simulink model "RBFNN_1221"  (R2018a)
settings: Solver=FixedStepAuto  StartTime=0.0  StopTime=inf  FixedStep=0.001  RelTol=1e-3  EnableMultiTasking=on
undefined symbols (not defined in the file): HIL, j, qc_get_step_size
libraries: dsparch4 x28, quarc_library x17, simulink x7, vrlib x1
(part 3 of 6)

== matlab function RBFNN_1221/MATLAB Function7 ==
  data: p_end input; s output; v_max input; a_max input; ts input; t input; v output; a output; j output
function [s, v, a, j] = fcn(p_end, v_max, a_max, ts, t)
y=[0,0,0,0];

v_M=v_max;
a_M=a_max;

j_M	  = a_M*20.0;  % Max jerk (the rate of acceleration) is set as 20*Max acceleration */
delay = 3;       %output trajectory is set as zero in the peroid of delay */
freq  = 1.0/ts;    %sampling frequency/
pause =1;		%when the trajectory moves to zero position and final position, pause 1 sec */


% compute initial condition of each trajectory segment */
t0  = pause;
t1  = a_M/j_M; %加速度增大
t2  = v_M/a_M - a_M/j_M;%加速度不变
t3  = a_M/j_M;

a1 = j_M*t1;
a2 = a1;
a3 = a2 - j_M*t3;

v1 = j_M*t1*t1/2.0;
v2 = v1 + a1*t2;
v3 = v2 + a2*t3 - j_M*t3*t3/2.0;

s1 = j_M*t1*t1*t1/6;
s2 = s1 + v1*t2 + a1*t2*t2/2.0;
s3 = s2 + v2*t3 + a2*t3*t3/2.0 - j_M*t3*t3*t3/6.0;

t4  = (p_end - 2.0*s3)/v_M;
t5  = a_M/j_M;
t6  = v_M/a_M - a_M/j_M;
t7  = a_M/j_M;
t8  = pause;
t9  = pause;
t10 = a_M/j_M;
t11 = v_M/a_M - a_M/j_M;
t12 = a_M/j_M;
t13 = (p_end - 2.0*s3)/v_M;
t14 = a_M/j_M;
t15 = v_M/a_M - a_M/j_M;
t16 = a_M/j_M;
t17 = pause;

a4  = a3;
a5  = a4 - j_M*t5;
a6  = a5;
a7  = a6 + j_M*t7;
a8  = a7;
a9  = a8;
a10 = a9 - j_M*t10;
a11 = a10;
a12 = a11 + j_M*t12;
a13 = a12;
a14 = a13 + j_M*t14;
a15 = a14;

v4  = v3 + a3*t4;
v5  = v4 + a4*t5 - j_M*t5*t5/2.0;
v6  = v5 + a5*t6;
v7  = v6 + a6*t7 + j_M*t7*t7/2.0;
v8  = v7 + a7*t8;
v9  = v8 + a8*t9;
v10 = v9 + a9*t10 - j_M*t10*t10/2.0;
v11 = v10 + a10*t11;
v12 = v11 + a11*t12 + j_M*t12*t12/2.0;
v13 = v12 + a12*t13;
v14 = v13 + a13*t14 + j_M*t14*t14/2.0;
v15 = v14 + a14*t15;

s4  = s3 + v3*t4 + a3*t4*t4/2.0;
s5  = s4 + v4*t5 + a4*t5*t5/2.0 - j_M*t5*t5*t5/6.0;
s6  = s5 + v5*t6 + a5*t6*t6/2.0;
s7  = s6 + v6*t7 + a6*t7*t7/2.0 + j_M*t7*t7*t7/6.0;
s8  = s7 + v7*t8 + a7*t8*t8/2.0;
s9  = s8 + v8*t9 + a8*t9*t9/2.0;
s10 = s9 + v9*t10 + a9*t10*t10/2.0 - j_M*t10*t10*t10/6.0;
s11 = s10 + v10*t11 + a10*t11*t11/2.0;
s12 = s11 + v11*t12 + a11*t12*t12/2.0 + j_M*t12*t12*t12/6.0;
s13 = s12 + v12*t13 + a12*t13*t13/2.0;
s14 = s13 + v13*t14 + a13*t14*t14/2.0 + j_M*t14*t14*t14/6.0;
s15 = s14 + v14*t15 + a14*t15*t15/2.0;
s16 = s15 + v15*t16 + a15*t16*t16/2.0 - j_M*t16*t16*t16/6.0;

T0  = t0;
T1  = T0 + t1;
T2  = T1 + t2;
T3  = T2 + t3;
T4  = T3 + t4;
T5  = T4 + t5;
T6  = T5 + t6;
T7  = T6 + t7;
T8  = T7 + t8;
T9  = T8 + t9;
T10 = T9 + t10;
T11 = T10 + t11;
T12 = T11 + t12;
T13 = T12 + t13;
T14 = T13 + t14;
T15 = T14 + t15;
T16 = T15 + t16;
T17 = T16 + t17;

%/* generate trajectory */
if(t<=delay)
    y(4) = 0.0;	   % /* jerk */
    y(2) = 0.0;		%/* acceleration */
    y(3) = 0.0;		%/* velocity */
    y(1) = 0.0;		%/* position */
else
    % 	 q0	  = *uPtrs[0];%q0 is what?
    T	  = T17*freq;
    tt   = (t-delay)*freq;
    rt   = mod(tt,T);
    rrt  = rt/freq;
    
    if(rt<=T0*freq)
        y(4) = 0.0;	   % /* jerk */
        y(3) = 0.0;		%/* acceleration */
        y(2) = 0.0;		%/* velocity */
        y(1) = 0.0;		%/* position */
    end
    
    if(rt>T0*freq && rt<=T1*freq)
        y(4) = j_M;
        y(3) = j_M*(rrt-T0);
        y(2) = j_M*(rrt-T0)*(rrt-T0)/2.0;
        y(1) = j_M*(rrt-T0)*(rrt-T0)*(rrt-T0)/6.0;
    end
    
    
    if(rt>T1*freq && rt<=T2*freq)
        y(4) = 0.0;
        y(3) = a1;
        y(2) = v1 + a1*(rrt-T1);
        y(1) = s1 + v1*(rrt-T1) + a1*(rrt-T1)*(rrt-T1)/2.0;
    end
    
    
    if(rt>T2*freq && rt<=T3*freq)
        y(4) = -j_M;
        y(3) = a2 - j_M*(rrt-T2);
        y(2) = v2 + a2*(rrt-T2) - j_M*(rrt-T2)*(rrt-T2)/2.0;
        y(1) = s2 + v2*(rrt-T2) + a2*(rrt-T2)*(rrt-T2)/2.0 - j_M*(rrt-T2)*(rrt-T2)*(rrt-T2)/6.0;
    end
    
    
    if(rt>T3*freq && rt<=T4*freq)
        y(4) = 0.0;
        y(3) = a3;
        y(2) = v3 + a3*(rrt-T3);
        y(1) = s3 + v3*(rrt-T3) + a3*(rrt-T3)*(rrt-T3)/2.0;
    end
    
    
    if(rt>T4*freq && rt<=T5*freq)
        y(4) = -j_M;
        y(3) = a4 - j_M*(rrt-T4);
        y(2) = v4 + a4*(rrt-T4) - j_M*(rrt-T4)*(rrt-T4)/2.0;
        y(1) = s4 + v4*(rrt-T4) + a4*(rrt-T4)*(rrt-T4)/2.0 - j_M*(rrt-T4)*(rrt-T4)*(rrt-T4)/6.0;
    end
    
    
    if(rt>T5*freq && rt<=T6*freq)
        y(4) = 0;
        y(3) = a5;
        y(2) = v5 + a5*(rrt-T5);
        y(1) = s5 + v5*(rrt-T5) + a5*(rrt-T5)*(rrt-T5)/2.0;
    end
    
    
    if(rt>T6*freq && rt<=T7*freq)
        y(4) = j_M;
        y(3) = a6 + j_M*(rrt-T6);
        y(2) = v6 + a6*(rrt-T6) + j_M*(rrt-T6)*(rrt-T6)/2.0;
        y(1) = s6 + v6*(rrt-T6) + a6*(rrt-T6)*(rrt-T6)/2.0 + j_M*(rrt-T6)*(rrt-T6)*(rrt-T6)/6.0;
    end
    
    
    if(rt>T7*freq && rt<=T8*freq)
        y(4) = 0.0;
        y(3) = 0.0;
        y(2) = 0.0;
        y(1) = s7;
    end
    
    
    if(rt>T8*freq && rt<=T9*freq)
        y(4) = 0.0;
        y(3) = 0.0;
        y(2) = 0.0;
        y(1) = s8;
    end
    
    
    if(rt>T9*freq && rt<=T10*freq)
        y(4) = -j_M;
        y(3) = a9 - j_M*(rrt-T9);
        y(2) = v9 + a9*(rrt-T9) - j_M*(rrt-T9)*(rrt-T9)/2.0;
        y(1) = s9 + v9*(rrt-T9) + a9*(rrt-T9)*(rrt-T9)/2.0 - j_M*(rrt-T9)*(rrt-T9)*(rrt-T9)/6.0;
    end
    
    
    if(rt>T10*freq && rt<=T11*freq)
        y(4) = 0.0;
        y(3) = a10;
        y(2) = v10 + a10*(rrt-T10);
        y(1) = s10 + v10*(rrt-T10) + a10*(rrt-T10)*(rrt-T10)/2.0;
    end
    
    
    
    if(rt>T11*freq && rt<=T12*freq)
        y(4) = j_M;
        y(3) = a11 + j_M*(rrt-T11);
        y(2) = v11 + a11*(rrt-T11) + j_M*(rrt-T11)*(rrt-T11)/2.0;
        y(1) = s11 + v11*(rrt-T11) + a11*(rrt-T11)*(rrt-T11)/2.0 + j_M*(rrt-T11)*(rrt-T11)*(rrt-T11)/6.0;
    end
    
    
    if(rt>T12*freq && rt<=T13*freq)
        y(4) = 0;
        y(3) = a12;
        y(2) = v12 + a12*(rrt-T12);
        y(1) = s12 + v12*(rrt-T12) + a12*(rrt-T12)*(rrt-T12)/2.0;
    end
    
    
    if(rt>T13*freq && rt<=T14*freq)
        y(4) = j_M;
        y(3) = a13 + j_M*(rrt-T13);
        y(2) = v13 + a13*(rrt-T13) + j_M*(rrt-T13)*(rrt-T13)/2.0;
        y(1) = s13 + v13*(rrt-T13) + a13*(rrt-T13)*(rrt-T13)/2.0 + j_M*(rrt-T13)*(rrt-T13)*(rrt-T13)/6.0;
    end
    
    
    if(rt>T14*freq && rt<=T15*freq)
        y(4) = 0.0;
        y(3) = a14;
        y(2) = v14 + a14*(rrt-T14);
        y(1) = s14 + v14*(rrt-T14) + a14*(rrt-T14)*(rrt-T14)/2.0;
    end
    
    
    if(rt>T15*freq && rt<=T16*freq)
        y(4) = -j_M;
        y(3) = a15 - j_M*(rrt-T15);
        y(2) = v15 + a15*(rrt-T15) - j_M*(rrt-T15)*(rrt-T15)/2.0;
        y(1) = s15 + v15*(rrt-T15) + a15*(rrt-T15)*(rrt-T15)/2.0 - j_M*(rrt-T15)*(rrt-T15)*(rrt-T15)/6.0;
    end
    
    
    if(rt>T16*freq && rt<=T17*freq)
        y(4) = 0.0;
        y(3) = 0.0;
        y(2) = 0.0;
        y(1) = s16;
    end
end
s = y(1);
v = y(2);
a = y(3);
j = y(4);

== matlab function RBFNN_1221/Obs Para Generator3 ==
  data: a input; gain input; k_obs output; th input
function k_obs = fcn(a, gain, th)

if a <= th
    b = 22.5*a-37.5;
else
    b = 31.16*a - 68.8; % a>=2.5
end
k_obs  = ([1 1/a 1/b] .* gain.^[1 2 3])';

== matlab function RBFNN_1221/Subsystem9/MATLAB Function1 ==
  data: x input; u input; y output
function y = fcn(x,u)
y=u(x);
end

== matlab function RBFNN_1221/MATLAB Function8 ==
  data: p_end input; s output; v_max input; a_max input; ts input; t input; v output; a output; j output
function [s, v, a, j] = fcn(p_end, v_max, a_max, ts, t)
y=[0,0,0,0];

v_M=v_max;
a_M=a_max;

j_M	  = a_M*20.0;  % Max jerk (the rate of acceleration) is set as 20*Max acceleration */
delay = 3;       %output trajectory is set as zero in the peroid of delay */
freq  = 1.0/ts;    %sampling frequency/
pause =1;		%when the trajectory moves to zero position and final position, pause 1 sec */


% compute initial condition of each trajectory segment */
t0  = pause;
t1  = a_M/j_M; %加速度增大
t2  = v_M/a_M - a_M/j_M;%加速度不变
t3  = a_M/j_M;

a1 = j_M*t1;
a2 = a1;
a3 = a2 - j_M*t3;

v1 = j_M*t1*t1/2.0;
v2 = v1 + a1*t2;
v3 = v2 + a2*t3 - j_M*t3*t3/2.0;

s1 = j_M*t1*t1*t1/6;
s2 = s1 + v1*t2 + a1*t2*t2/2.0;
s3 = s2 + v2*t3 + a2*t3*t3/2.0 - j_M*t3*t3*t3/6.0;

t4  = (p_end - 2.0*s3)/v_M;
t5  = a_M/j_M;
t6  = v_M/a_M - a_M/j_M;
t7  = a_M/j_M;
t8  = pause;
t9  = pause;
t10 = a_M/j_M;
t11 = v_M/a_M - a_M/j_M;
t12 = a_M/j_M;
t13 = (p_end - 2.0*s3)/v_M;
t14 = a_M/j_M;
t15 = v_M/a_M - a_M/j_M;
t16 = a_M/j_M;
t17 = pause;

a4  = a3;
a5  = a4 - j_M*t5;
a6  = a5;
a7  = a6 + j_M*t7;
a8  = a7;
a9  = a8;
a10 = a9 - j_M*t10;
a11 = a10;
a12 = a11 + j_M*t12;
a13 = a12;
a14 = a13 + j_M*t14;
a15 = a14;

v4  = v3 + a3*t4;
v5  = v4 + a4*t5 - j_M*t5*t5/2.0;
v6  = v5 + a5*t6;
v7  = v6 + a6*t7 + j_M*t7*t7/2.0;
v8  = v7 + a7*t8;
v9  = v8 + a8*t9;
v10 = v9 + a9*t10 - j_M*t10*t10/2.0;
v11 = v10 + a10*t11;
v12 = v11 + a11*t12 + j_M*t12*t12/2.0;
v13 = v12 + a12*t13;
v14 = v13 + a13*t14 + j_M*t14*t14/2.0;
v15 = v14 + a14*t15;

s4  = s3 + v3*t4 + a3*t4*t4/2.0;
s5  = s4 + v4*t5 + a4*t5*t5/2.0 - j_M*t5*t5*t5/6.0;
s6  = s5 + v5*t6 + a5*t6*t6/2.0;
s7  = s6 + v6*t7 + a6*t7*t7/2.0 + j_M*t7*t7*t7/6.0;
s8  = s7 + v7*t8 + a7*t8*t8/2.0;
s9  = s8 + v8*t9 + a8*t9*t9/2.0;
s10 = s9 + v9*t10 + a9*t10*t10/2.0 - j_M*t10*t10*t10/6.0;
s11 = s10 + v10*t11 + a10*t11*t11/2.0;
s12 = s11 + v11*t12 + a11*t12*t12/2.0 + j_M*t12*t12*t12/6.0;
s13 = s12 + v12*t13 + a12*t13*t13/2.0;
s14 = s13 + v13*t14 + a13*t14*t14/2.0 + j_M*t14*t14*t14/6.0;
s15 = s14 + v14*t15 + a14*t15*t15/2.0;
s16 = s15 + v15*t16 + a15*t16*t16/2.0 - j_M*t16*t16*t16/6.0;

T0  = t0;
T1  = T0 + t1;
T2  = T1 + t2;
T3  = T2 + t3;
T4  = T3 + t4;
T5  = T4 + t5;
T6  = T5 + t6;
T7  = T6 + t7;
T8  = T7 + t8;
T9  = T8 + t9;
T10 = T9 + t10;
T11 = T10 + t11;
T12 = T11 + t12;
T13 = T12 + t13;
T14 = T13 + t14;
T15 = T14 + t15;
T16 = T15 + t16;
T17 = T16 + t17;

%/* generate trajectory */
if(t<=delay)
    y(4) = 0.0;	   % /* jerk */
    y(2) = 0.0;		%/* acceleration */
    y(3) = 0.0;		%/* velocity */
    y(1) = 0.0;		%/* position */
else
    % 	 q0	  = *uPtrs[0];%q0 is what?
    T	  = T17*freq;
    tt   = (t-delay)*freq;
    rt   = mod(tt,T);
    rrt  = rt/freq;
    
    if(rt<=T0*freq)
        y(4) = 0.0;	   % /* jerk */
        y(3) = 0.0;		%/* acceleration */
        y(2) = 0.0;		%/* velocity */
        y(1) = 0.0;		%/* position */
    end
    
    if(rt>T0*freq && rt<=T1*freq)
        y(4) = j_M;
        y(3) = j_M*(rrt-T0);
        y(2) = j_M*(rrt-T0)*(rrt-T0)/2.0;
        y(1) = j_M*(rrt-T0)*(rrt-T0)*(rrt-T0)/6.0;
    end
    
    
    if(rt>T1*freq && rt<=T2*freq)
        y(4) = 0.0;
        y(3) = a1;
        y(2) = v1 + a1*(rrt-T1);
        y(1) = s1 + v1*(rrt-T1) + a1*(rrt-T1)*(rrt-T1)/2.0;
    end
    
    
    if(rt>T2*freq && rt<=T3*freq)
        y(4) = -j_M;
        y(3) = a2 - j_M*(rrt-T2);
        y(2) = v2 + a2*(rrt-T2) - j_M*(rrt-T2)*(rrt-T2)/2.0;
        y(1) = s2 + v2*(rrt-T2) + a2*(rrt-T2)*(rrt-T2)/2.0 - j_M*(rrt-T2)*(rrt-T2)*(rrt-T2)/6.0;
    end
    
    
    if(rt>T3*freq && rt<=T4*freq)
        y(4) = 0.0;
        y(3) = a3;
        y(2) = v3 + a3*(rrt-T3);
        y(1) = s3 + v3*(rrt-T3) + a3*(rrt-T3)*(rrt-T3)/2.0;
    end
    
    
    if(rt>T4*freq && rt<=T5*freq)
        y(4) = -j_M;
        y(3) = a4 - j_M*(rrt-T4);
        y(2) = v4 + a4*(rrt-T4) - j_M*(rrt-T4)*(rrt-T4)/2.0;
        y(1) = s4 + v4*(rrt-T4) + a4*(rrt-T4)*(rrt-T4)/2.0 - j_M*(rrt-T4)*(rrt-T4)*(rrt-T4)/6.0;
    end
    
    
    if(rt>T5*freq && rt<=T6*freq)
        y(4) = 0;
        y(3) = a5;
        y(2) = v5 + a5*(rrt-T5);
        y(1) = s5 + v5*(rrt-T5) + a5*(rrt-T5)*(rrt-T5)/2.0;
    end
    
    
    if(rt>T6*freq && rt<=T7*freq)
        y(4) = j_M;
        y(3) = a6 + j_M*(rrt-T6);
        y(2) = v6 + a6*(rrt-T6) + j_M*(rrt-T6)*(rrt-T6)/2.0;
        y(1) = s6 + v6*(rrt-T6) + a6*(rrt-T6)*(rrt-T6)/2.0 + j_M*(rrt-T6)*(rrt-T6)*(rrt-T6)/6.0;
    end
    
    
    if(rt>T7*freq && rt<=T8*freq)
        y(4) = 0.0;
        y(3) = 0.0;
        y(2) = 0.0;
        y(1) = s7;
    end
    
    
    if(rt>T8*freq && rt<=T9*freq)
        y(4) = 0.0;
        y(3) = 0.0;
        y(2) = 0.0;
        y(1) = s8;
    end
    
    
    if(rt>T9*freq && rt<=T10*freq)
        y(4) = -j_M;
        y(3) = a9 - j_M*(rrt-T9);
        y(2) = v9 + a9*(rrt-T9) - j_M*(rrt-T9)*(rrt-T9)/2.0;
        y(1) = s9 + v9*(rrt-T9) + a9*(rrt-T9)*(rrt-T9)/2.0 - j_M*(rrt-T9)*(rrt-T9)*(rrt-T9)/6.0;
    end
    
    
    if(rt>T10*freq && rt<=T11*freq)
        y(4) = 0.0;
        y(3) = a10;
        y(2) = v10 + a10*(rrt-T10);
        y(1) = s10 + v10*(rrt-T10) + a10*(rrt-T10)*(rrt-T10)/2.0;
    end
    
    
    
    if(rt>T11*freq && rt<=T12*freq)
        y(4) = j_M;
        y(3) = a11 + j_M*(rrt-T11);
        y(2) = v11 + a11*(rrt-T11) + j_M*(rrt-T11)*(rrt-T11)/2.0;
        y(1) = s11 + v11*(rrt-T11) + a11*(rrt-T11)*(rrt-T11)/2.0 + j_M*(rrt-T11)*(rrt-T11)*(rrt-T11)/6.0;
    end
    
    
    if(rt>T12*freq && rt<=T13*freq)
        y(4) = 0;
        y(3) = a12;
        y(2) = v12 + a12*(rrt-T12);
        y(1) = s12 + v12*(rrt-T12) + a12*(rrt-T12)*(rrt-T12)/2.0;
    end
    
    
    if(rt>T13*freq && rt<=T14*freq)
        y(4) = j_M;
        y(3) = a13 + j_M*(rrt-T13);
        y(2) = v13 + a13*(rrt-T13) + j_M*(rrt-T13)*(rrt-T13)/2.0;
        y(1) = s13 + v13*(rrt-T13) + a13*(rrt-T13)*(rrt-T13)/2.0 + j_M*(rrt-T13)*(rrt-T13)*(rrt-T13)/6.0;
    end
    
    
    if(rt>T14*freq && rt<=T15*freq)
        y(4) = 0.0;
        y(3) = a14;
        y(2) = v14 + a14*(rrt-T14);
        y(1) = s14 + v14*(rrt-T14) + a14*(rrt-T14)*(rrt-T14)/2.0;
    end
    
    
    if(rt>T15*freq && rt<=T16*freq)
        y(4) = -j_M;
        y(3) = a15 - j_M*(rrt-T15);
        y(2) = v15 + a15*(rrt-T15) - j_M*(rrt-T15)*(rrt-T15)/2.0;
        y(1) = s15 + v15*(rrt-T15) + a15*(rrt-T15)*(rrt-T15)/2.0 - j_M*(rrt-T15)*(rrt-T15)*(rrt-T15)/6.0;
    end
    
    
    if(rt>T16*freq && rt<=T17*freq)
        y(4) = 0.0;
        y(3) = 0.0;
        y(2) = 0.0;
        y(1) = s16;
    end
end
s = y(1);
v = y(2);
a = y(3);
j = y(4);

== matlab function RBFNN_1221/limit_u2 ==
  data: u input; y output
function y = fcn(u)
y=u;
if u>10
    y=10;
end
if u<-10
    y=-10;
end
end

== matlab function RBFNN_1221/MATLAB Function1 ==
  data: bias input; out output; xv input
function out = fcn(bias,xv)
out = xv;
if xv > 0
    out = xv + bias;
end
if xv < 0
    out = xv - bias;
end
end

== matlab function RBFNN_1221/Obs Para Generator4 ==
  data: a input; gain input; k_obs output; th input
function k_obs = fcn(a, gain, th)

if a <= th
    b = 22.5*a-37.5;
else
    b = 31.16*a - 68.8; % a>=2.5
end
k_obs  = ([1 1/a 1/b] .* gain.^[1 2 3])';

== matlab function RBFNN_1221/MATLAB Function9 ==
  data: p_end input; s output; v_max input; a_max input; ts input; t input; v output; a output; j output
function [s, v, a, j] = fcn(p_end, v_max, a_max, ts, t)
y=[0,0,0,0];

v_M=v_max;
a_M=a_max;

j_M	  = a_M*20.0;  % Max jerk (the rate of acceleration) is set as 20*Max acceleration */
delay = 3;       %output trajectory is set as zero in the peroid of delay */
freq  = 1.0/ts;    %sampling frequency/
pause =1;		%when the trajectory moves to zero position and final position, pause 1 sec */


% compute initial condition of each trajectory segment */
t0  = pause;
t1  = a_M/j_M; %加速度增大
t2  = v_M/a_M - a_M/j_M;%加速度不变
t3  = a_M/j_M;

a1 = j_M*t1;
a2 = a1;
a3 = a2 - j_M*t3;

v1 = j_M*t1*t1/2.0;
v2 = v1 + a1*t2;
v3 = v2 + a2*t3 - j_M*t3*t3/2.0;

s1 = j_M*t1*t1*t1/6;
s2 = s1 + v1*t2 + a1*t2*t2/2.0;
s3 = s2 + v2*t3 + a2*t3*t3/2.0 - j_M*t3*t3*t3/6.0;

t4  = (p_end - 2.0*s3)/v_M;
t5  = a_M/j_M;
t6  = v_M/a_M - a_M/j_M;
t7  = a_M/j_M;
t8  = pause;
t9  = pause;
t10 = a_M/j_M;
t11 = v_M/a_M - a_M/j_M;
t12 = a_M/j_M;
t13 = (p_end - 2.0*s3)/v_M;
t14 = a_M/j_M;
t15 = v_M/a_M - a_M/j_M;
t16 = a_M/j_M;
t17 = pause;

a4  = a3;
a5  = a4 - j_M*t5;
a6  = a5;
a7  = a6 + j_M*t7;
a8  = a7;
a9  = a8;
a10 = a9 - j_M*t10;
a11 = a10;
a12 = a11 + j_M*t12;
a13 = a12;
a14 = a13 + j_M*t14;
a15 = a14;

v4  = v3 + a3*t4;
v5  = v4 + a4*t5 - j_M*t5*t5/2.0;
v6  = v5 + a5*t6;
v7  = v6 + a6*t7 + j_M*t7*t7/2.0;
v8  = v7 + a7*t8;
v9  = v8 + a8*t9;
v10 = v9 + a9*t10 - j_M*t10*t10/2.0;
v11 = v10 + a10*t11;
v12 = v11 + a11*t12 + j_M*t12*t12/2.0;
v13 = v12 + a12*t13;
v14 = v13 + a13*t14 + j_M*t14*t14/2.0;
v15 = v14 + a14*t15;

s4  = s3 + v3*t4 + a3*t4*t4/2.0;
s5  = s4 + v4*t5 + a4*t5*t5/2.0 - j_M*t5*t5*t5/6.0;
s6  = s5 + v5*t6 + a5*t6*t6/2.0;
s7  = s6 + v6*t7 + a6*t7*t7/2.0 + j_M*t7*t7*t7/6.0;
s8  = s7 + v7*t8 + a7*t8*t8/2.0;
s9  = s8 + v8*t9 + a8*t9*t9/2.0;
s10 = s9 + v9*t10 + a9*t10*t10/2.0 - j_M*t10*t10*t10/6.0;
s11 = s10 + v10*t11 + a10*t11*t11/2.0;
s12 = s11 + v11*t12 + a11*t12*t12/2.0 + j_M*t12*t12*t12/6.0;
s13 = s12 + v12*t13 + a12*t13*t13/2.0;
s14 = s13 + v13*t14 + a13*t14*t14/2.0 + j_M*t14*t14*t14/6.0;
s15 = s14 + v14*t15 + a14*t15*t15/2.0;
s16 = s15 + v15*t16 + a15*t16*t16/2.0 - j_M*t16*t16*t16/6.0;

T0  = t0;
T1  = T0 + t1;
T2  = T1 + t2;
T3  = T2 + t3;
T4  = T3 + t4;
T5  = T4 + t5;
T6  = T5 + t6;
T7  = T6 + t7;
T8  = T7 + t8;
T9  = T8 + t9;
T10 = T9 + t10;
T11 = T10 + t11;
T12 = T11 + t12;
T13 = T12 + t13;
T14 = T13 + t14;
T15 = T14 + t15;
T16 = T15 + t16;
T17 = T16 + t17;

%/* generate trajectory */
if(t<=delay)
    y(4) = 0.0;	   % /* jerk */
    y(2) = 0.0;		%/* acceleration */
    y(3) = 0.0;		%/* velocity */
    y(1) = 0.0;		%/* position */
else
    % 	 q0	  = *uPtrs[0];%q0 is what?
    T	  = T17*freq;
    tt   = (t-delay)*freq;
    rt   = mod(tt,T);
    rrt  = rt/freq;
    
    if(rt<=T0*freq)
        y(4) = 0.0;	   % /* jerk */
        y(3) = 0.0;		%/* acceleration */
        y(2) = 0.0;		%/* velocity */
        y(1) = 0.0;		%/* position */
    end
    
    if(rt>T0*freq && rt<=T1*freq)
        y(4) = j_M;
        y(3) = j_M*(rrt-T0);
        y(2) = j_M*(rrt-T0)*(rrt-T0)/2.0;
        y(1) = j_M*(rrt-T0)*(rrt-T0)*(rrt-T0)/6.0;
    end
    
    
    if(rt>T1*freq && rt<=T2*freq)
        y(4) = 0.0;
        y(3) = a1;
        y(2) = v1 + a1*(rrt-T1);
        y(1) = s1 + v1*(rrt-T1) + a1*(rrt-T1)*(rrt-T1)/2.0;
    end
    
    
    if(rt>T2*freq && rt<=T3*freq)
        y(4) = -j_M;
        y(3) = a2 - j_M*(rrt-T2);
        y(2) = v2 + a2*(rrt-T2) - j_M*(rrt-T2)*(rrt-T2)/2.0;
        y(1) = s2 + v2*(rrt-T2) + a2*(rrt-T2)*(rrt-T2)/2.0 - j_M*(rrt-T2)*(rrt-T2)*(rrt-T2)/6.0;
    end
    
    
    if(rt>T3*freq && rt<=T4*freq)
        y(4) = 0.0;
        y(3) = a3;
        y(2) = v3 + a3*(rrt-T3);
        y(1) = s3 + v3*(rrt-T3) + a3*(rrt-T3)*(rrt-T3)/2.0;
    end
    
    
    if(rt>T4*freq && rt<=T5*freq)
        y(4) = -j_M;
        y(3) = a4 - j_M*(rrt-T4);
        y(2) = v4 + a4*(rrt-T4) - j_M*(rrt-T4)*(rrt-T4)/2.0;
        y(1) = s4 + v4*(rrt-T4) + a4*(rrt-T4)*(rrt-T4)/2.0 - j_M*(rrt-T4)*(rrt-T4)*(rrt-T4)/6.0;
    end
    
    
    if(rt>T5*freq && rt<=T6*freq)
        y(4) = 0;
        y(3) = a5;
        y(2) = v5 + a5*(rrt-T5);
        y(1) = s5 + v5*(rrt-T5) + a5*(rrt-T5)*(rrt-T5)/2.0;
    end
    
    
    if(rt>T6*freq && rt<=T7*freq)
        y(4) = j_M;
        y(3) = a6 + j_M*(rrt-T6);
        y(2) = v6 + a6*(rrt-T6) + j_M*(rrt-T6)*(rrt-T6)/2.0;
        y(1) = s6 + v6*(rrt-T6) + a6*(rrt-T6)*(rrt-T6)/2.0 + j_M*(rrt-T6)*(rrt-T6)*(rrt-T6)/6.0;
    end
    
    
    if(rt>T7*freq && rt<=T8*freq)
        y(4) = 0.0;
        y(3) = 0.0;
        y(2) = 0.0;
        y(1) = s7;
    end
    
    
    if(rt>T8*freq && rt<=T9*freq)
        y(4) = 0.0;
        y(3) = 0.0;
        y(2) = 0.0;
        y(1) = s8;
    end
    
    
    if(rt>T9*freq && rt<=T10*freq)
        y(4) = -j_M;
        y(3) = a9 - j_M*(rrt-T9);
        y(2) = v9 + a9*(rrt-T9) - j_M*(rrt-T9)*(rrt-T9)/2.0;
        y(1) = s9 + v9*(rrt-T9) + a9*(rrt-T9)*(rrt-T9)/2.0 - j_M*(rrt-T9)*(rrt-T9)*(rrt-T9)/6.0;
    end
    
    
    if(rt>T10*freq && rt<=T11*freq)
        y(4) = 0.0;
        y(3) = a10;
        y(2) = v10 + a10*(rrt-T10);
        y(1) = s10 + v10*(rrt-T10) + a10*(rrt-T10)*(rrt-T10)/2.0;
    end
    
    
    
    if(rt>T11*freq && rt<=T12*freq)
        y(4) = j_M;
        y(3) = a11 + j_M*(rrt-T11);
        y(2) = v11 + a11*(rrt-T11) + j_M*(rrt-T11)*(rrt-T11)/2.0;
        y(1) = s11 + v11*(rrt-T11) + a11*(rrt-T11)*(rrt-T11)/2.0 + j_M*(rrt-T11)*(rrt-T11)*(rrt-T11)/6.0;
    end
    
    
    if(rt>T12*freq && rt<=T13*freq)
        y(4) = 0;
        y(3) = a12;
        y(2) = v12 + a12*(rrt-T12);
        y(1) = s12 + v12*(rrt-T12) + a12*(rrt-T12)*(rrt-T12)/2.0;
    end
    
    
    if(rt>T13*freq && rt<=T14*freq)
        y(4) = j_M;
        y(3) = a13 + j_M*(rrt-T13);
        y(2) = v13 + a13*(rrt-T13) + j_M*(rrt-T13)*(rrt-T13)/2.0;
        y(1) = s13 + v13*(rrt-T13) + a13*(rrt-T13)*(rrt-T13)/2.0 + j_M*(rrt-T13)*(rrt-T13)*(rrt-T13)/6.0;
    end
    
    
    if(rt>T14*freq && rt<=T15*freq)
        y(4) = 0.0;
        y(3) = a14;
        y(2) = v14 + a14*(rrt-T14);
        y(1) = s14 + v14*(rrt-T14) + a14*(rrt-T14)*(rrt-T14)/2.0;
    end
    
    
    if(rt>T15*freq && rt<=T16*freq)
        y(4) = -j_M;
        y(3) = a15 - j_M*(rrt-T15);
        y(2) = v15 + a15*(rrt-T15) - j_M*(rrt-T15)*(rrt-T15)/2.0;
        y(1) = s15 + v15*(rrt-T15) + a15*(rrt-T15)*(rrt-T15)/2.0 - j_M*(rrt-T15)*(rrt-T15)*(rrt-T15)/6.0;
    end
    
    
    if(rt>T16*freq && rt<=T17*freq)
        y(4) = 0.0;
        y(3) = 0.0;
        y(2) = 0.0;
        y(1) = s16;
    end
end
s = y(1);
v = y(2);
a = y(3);
j = y(4);

== matlab function RBFNN_1221/limit_u3 ==
  data: u input; y output
function y = fcn(u)
y=u;
if u>10
    y=10;
end
if u<-10
    y=-10;
end
end

== matlab function RBFNN_1221/Subsystem8/Enabled Subsystem/Round Traj Planner ==
  data: p_center input; p_round output size=[3,1]; v_normal input; radius input; theta input; v_toward input; q_round output size=[4 1]; err output size=1
function [p_round, q_round, err] = fcn(p_center, v_normal, radius, theta, v_toward)

temp = atan2(-v_normal(3),v_normal(1));
v_init_r = [sin(temp),0,cos(temp)];
v_orth = cross(v_normal, v_init_r);
p_round = p_center + radius * (v_init_r'.*cos(theta) + v_orth.'*sin(theta));
q_round = InvKin(v_toward, p_round);

err = 0;
if max(abs(imag(q_round))~=0)
	err = err+1;
elseif isnan(sum(q_round))
	err = err+2;
end

== matlab function RBFNN_1221/Subsystem9/MATLAB Function ==
  data: Xcenter input; Ycenter input; height1 input; traj output size=[1 3]; height2 input; scale_factor input; span input; phase input; phase_last input; phase_start_time_last input; time input; phase_start_time output; err output
% ZJU形状轨迹生成
% 
% height1：书写高度
% height2：抬起高度

function [traj, phase_start_time, err] = fcn(Xcenter, Ycenter, height1, height2, scale_factor, span, phase, phase_last, phase_start_time_last, time)

% 平移缩放
% Traj_Z = [3.48433829875678,35.4885053891162;5.19457971416122,35.5831283413590;7.07593708942604,35.6227938555666;9.01422182304440,35.7222247489255;11.1233721029233,35.9423883858658;12.6056536713138,35.9736400031203;14.4300002170251,36.0121035320489;15.7412492967551,36.0397491934664;16.9954875469317,36.0661928696048;18.4209252281685,35.9791157138358;19.7320073654987,36.1238881629977;20.8151296558149,36.2052892771713;22.0122736052380,36.2890943619029;23.4945551736285,36.3203459791574;24.8628150829120,36.3491936258538;25.9460208444281,36.3720313461552;26.0030316739815,36.3732333314342;26.0030316739815,36.3732333314342;26.0030316739815,36.3732333314342;24.8647349205104,35.0022355667930;24.0114923148066,33.6372477285468;23.4995634456244,32.8065423468247;22.8165186165817,32.0307944031377;22.0201198980316,30.7841353379149;21.1101168763742,29.2422553327731;20.3141355138237,27.7027792981893;19.5175698528737,26.5732470207110;18.4365343425558,25.0277610597321;17.6400521528057,23.8396653883816;16.6725374743952,22.6479637611940;15.8192113974915,21.3415393168201;14.7375915887741,20.2059971129467;13.7698264967638,19.1899856673758;12.6312793296929,17.9946780843511;11.8923087966959,16.4564040350464;10.8106889879785,15.3208618311730;10.0138729134287,14.3670197353113;9.50202751544635,13.4777509597169;8.02174925585426,12.0409778895293;7.33953913881094,10.6795960071202;6.20132585653972,9.25003484860675;5.23439547652874,7.64838946431369;4.43791328677867,6.46029379296318;3.18551140300062,5.14545545163609;3.24293958855376,4.85384046755404;3.41405554841413,4.79888302951889;3.52807720752109,4.80128700007692;3.58508803707457,4.80248898535594;3.64209886662805,4.80369097063496;5.18130779337206,4.89470796704069;6.77744407846961,5.04549034259766;7.68953388012534,5.12328550093417;8.88659435834854,5.26565397953800;10.4828141146460,5.35787296122275;12.3069937179575,5.51346327789579;13.2762612915666,5.47533363376691;14.6445212008501,5.50418128046337;16.5826389920686,5.72073896156666;18.0651709740588,5.57630039720452;19.6614742015562,5.60995598501705;21.7137805942816,5.71179084893396;23.4808658968396,5.92474257420019;25.1914411970438,5.78511195095413;27.0157877427551,5.82357547988274;27.1296424594622,5.94310623818520;27.2439980033689,5.71125663325439];
% Traj_U = [72.6379737199274,37.2978938957997;72.5256214848191,36.1242220477974;72.5270404952180,35.1286443519698;72.4151056161093,33.6621555346065;72.2455756090476,32.6044084890696;72.5317148824142,31.8490942951259;72.4764569480592,30.6180610385304;72.4777924872581,29.6810467365751;72.4797123248566,28.3340886775142;72.4810478640555,27.3970743755588;72.4827172880541,26.2258064981145;72.4853883664519,24.3517778942037;72.5447363896035,22.7132048510608;72.7753673150153,20.9025475821383;72.7767863254142,19.9069698863107;72.8924774085198,18.7381059794245;72.8941468325184,17.5668381019802;72.8956493141172,16.5126970122804;73.0111734548229,15.4609598931386;73.4120021568958,14.2395425187753;73.6411306007089,13.4830263395526;74.0412915331823,12.7301161161670;74.4414524656558,11.9772058927814;75.0127293579896,11.1693382313606;75.5270788919699,10.3017051907886;75.9268224684437,9.84161193676402;76.9540190548055,9.16048694531982;77.8099327389071,8.65144617965519;78.6657629518088,8.20096880786279;79.4648327487567,7.57359926917472;80.4347680919653,7.06696247406814;81.5753185678346,6.85674860415967;82.2026881065226,6.69428026061224;83.2858938680387,6.71711798091361;84.3690996295549,6.73995570121497;85.6233378797314,6.76639937735339;87.3331619391362,7.15383929895724;88.9280461562348,8.18307258259739;89.8964790178445,8.73057687719062;90.5793569044873,9.62345160862204;91.6614775404043,10.4076134492622;92.7432642915215,11.4260288653911;93.0844945568431,12.0188747157874;93.5956721852260,13.3766506423594;93.5940862324273,14.4893551259315;93.5922498660288,15.7777497911201;93.6467565595843,17.5358535925655;93.7011797819399,19.3525207878831;93.6998442427410,20.2895350898385;93.6404962195894,21.9281081329814;93.6394945651902,22.6308688594480;93.5805638980383,23.9766249332299;93.6351540627938,25.6761653408030;93.5766407516415,26.7291044452238;93.6879078611507,28.6641004135649;93.6853202539528,30.4795656236035;93.6827326467549,32.2950308336420;93.8515948842171,33.8212850301566;93.8490072770192,35.6367502401952;93.9041817401742,36.9263468906629;94.0732943912362,38.2769109055608];
% Traj_J = [51.9417070528156,37.7985875414711;51.9234825074971,37.2515952035708;51.9052579621787,36.7046028656705;51.8870334168602,36.1576105277702;51.8310242417059,35.4536478160246;51.7750150665516,34.7496851042790;51.7190058913973,34.0457223925335;51.7196180135302,33.6162575041373;51.7202301356630,33.1867926157410;51.7208422577958,32.7573277273448;51.7786321518820,32.2119380364832;51.8364220459682,31.6665483456216;51.8942119400543,31.1211586547599;51.8381192937001,30.4757593368866;51.7820266473459,29.8303600190132;51.7259340009917,29.1849607011399;51.7650819937597,28.3853956417390;51.8042299865278,27.5858305823381;51.8433779792958,26.7862655229372;51.8252369051773,26.1807097911647;51.8070958310588,25.5751540593921;51.7889547569402,24.9695983276196;51.8280471022417,24.2090755308002;51.8671394475431,23.4485527339808;51.9062317928445,22.6880299371613;51.9259866434951,22.1613600540711;51.9457414941456,21.6346901709809;51.9654963447962,21.1080202878906;51.9663867042621,20.4833440865870;51.9672770637281,19.8586678852834;51.9681674231940,19.2339916839798;51.9690577826599,18.6093154826762;51.9699481421259,17.9846392813726;51.9708385015918,17.3599630800691;51.9716453898578,16.7938502726377;51.9724522781238,16.2277374652063;51.9732591663898,15.6616246577749;51.9175004048353,14.7819717644127;51.8617416432808,13.9023188710505;51.8059828817263,13.0226659776883;51.6930463482185,12.2589378867915;51.5801098147107,11.4952097958947;51.4671732812028,10.7314817049979;51.2590795797726,10.0633559617564;51.0509858783424,9.39523021851494;50.8428921769122,8.72710447527346;50.4444284921707,8.28922568992410;50.0459648074292,7.85134690457475;49.6475011226877,7.41346811922539;49.2677349867309,7.19072243983381;48.8879688507741,6.96797676044224;48.5082027148173,6.74523108105066;47.8244901161752,6.43799028834137;47.1407775175331,6.13074949563208;46.4570649188910,5.82350870292279;45.7160076058958,5.74931950042333;44.9749502929005,5.67513029792387;44.2338929799052,5.60094109542441;43.5876589500325,5.66540312075847;42.9414249201598,5.72986514609254;42.2951908902871,5.79432717142660;41.9719904041509,5.88512157796585;41.6487899180146,5.97591598450510;41.3255894318783,6.06671039104434;40.8692523818507,6.23278469042882;40.4129153318231,6.39885898981331;39.9565782817954,6.56493328919779];
Traj_Z = [3.48433829875678,35.4885053891162;5.19457971416122,35.5831283413590;7.07593708942604,35.6227938555666;9.01422182304440,35.7222247489255;11.1233721029233,35.9423883858658;12.6056536713138,35.9736400031203;14.4300002170251,36.0121035320489;15.7412492967551,36.0397491934664;16.9954875469317,36.0661928696048;18.4209252281685,35.9791157138358;19.7320073654987,36.1238881629977;20.8151296558149,36.2052892771713;22.0122736052380,36.2890943619029;23.4945551736285,36.3203459791574;24.8628150829120,36.3491936258538;25.9460208444281,36.3720313461552;26.0030316739815,36.3732333314342;26.0030316739815,36.3732333314342;26.0030316739815,36.3732333314342;26.0030316739815,36.3732333314342;26.0030316739815,36.3732333314342;26.0030316739815,36.3732333314342;26.0030316739815,36.3732333314342;26.0030316739815,36.3732333314342;26.0030316739815,36.3732333314342;26.0030316739815,36.3732333314342;26.0030316739815,36.3732333314342;24.8647349205104,35.0022355667930;24.0114923148066,33.6372477285468;23.4995634456244,32.8065423468247;22.8165186165817,32.0307944031377;22.0201198980316,30.7841353379149;21.1101168763742,29.2422553327731;20.3141355138237,27.7027792981893;19.5175698528737,26.5732470207110;18.4365343425558,25.0277610597321;17.6400521528057,23.8396653883816;16.6725374743952,22.6479637611940;15.8192113974915,21.3415393168201;14.7375915887741,20.2059971129467;13.7698264967638,19.1899856673758;12.6312793296929,17.9946780843511;11.8923087966959,16.4564040350464;10.8106889879785,15.3208618311730;10.0138729134287,14.3670197353113;9.50202751544635,13.4777509597169;8.02174925585426,12.0409778895293;7.33953913881094,10.6795960071202;6.20132585653972,9.25003484860675;5.23439547652874,7.64838946431369;4.43791328677867,6.46029379296318;3.18551140300062,5.14545545163609;3.18551140300062,5.14545545163609;3.18551140300062,5.14545545163609;3.18551140300062,5.14545545163609;3.18551140300062,5.14545545163609;3.18551140300062,5.14545545163609;3.18551140300062,5.14545545163609;3.18551140300062,5.14545545163609;3.24293958855376,4.85384046755404;3.41405554841413,4.79888302951889;3.52807720752109,4.80128700007692;3.58508803707457,4.80248898535594;3.64209886662805,4.80369097063496;5.18130779337206,4.89470796704069;6.77744407846961,5.04549034259766;7.68953388012534,5.12328550093417;8.88659435834854,5.26565397953800;10.4828141146460,5.35787296122275;12.3069937179575,5.51346327789579;13.2762612915666,5.47533363376691;14.6445212008501,5.50418128046337;16.5826389920686,5.72073896156666;18.0651709740588,5.57630039720452;19.6614742015562,5.60995598501705;21.7137805942816,5.71179084893396;23.4808658968396,5.92474257420019;25.1914411970438,5.78511195095413;27.0157877427551,5.82357547988274;27.1296424594622,5.94310623818520;27.2439980033689,5.71125663325439;27.2439980033689,5.71125663325439;27.2439980033689,5.71125663325439;27.2439980033689,5.71125663325439;27.2439980033689,5.71125663325439;27.2439980033689,5.71125663325439;27.2439980033689,5.71125663325439;27.2439980033689,5.71125663325439];
Traj_U = [72.6379737199274,37.2978938957997;72.6379737199274,37.2978938957997;72.6379737199274,37.2978938957997;72.6379737199274,37.2978938957997;72.6379737199274,37.2978938957997;72.6379737199274,37.2978938957997;72.5256214848191,36.1242220477974;72.5270404952180,35.1286443519698;72.4151056161093,33.6621555346065;72.2455756090476,32.6044084890696;72.5317148824142,31.8490942951259;72.4764569480592,30.6180610385304;72.4777924872581,29.6810467365751;72.4797123248566,28.3340886775142;72.4810478640555,27.3970743755588;72.4827172880541,26.2258064981145;72.4853883664519,24.3517778942037;72.5447363896035,22.7132048510608;72.7753673150153,20.9025475821383;72.7767863254142,19.9069698863107;72.8924774085198,18.7381059794245;72.8941468325184,17.5668381019802;72.8956493141172,16.5126970122804;73.0111734548229,15.4609598931386;73.4120021568958,14.2395425187753;73.6411306007089,13.4830263395526;74.0412915331823,12.7301161161670;74.4414524656558,11.9772058927814;75.0127293579896,11.1693382313606;75.5270788919699,10.3017051907886;75.9268224684437,9.84161193676402;76.9540190548055,9.16048694531982;77.8099327389071,8.65144617965519;78.6657629518088,8.20096880786279;79.4648327487567,7.57359926917472;80.4347680919653,7.06696247406814;81.5753185678346,6.85674860415967;82.2026881065226,6.69428026061224;83.2858938680387,6.71711798091361;84.3690996295549,6.73995570121497;85.6233378797314,6.76639937735339;87.3331619391362,7.15383929895724;88.9280461562348,8.18307258259739;89.8964790178445,8.73057687719062;90.5793569044873,9.62345160862204;91.6614775404043,10.4076134492622;92.7432642915215,11.4260288653911;93.0844945568431,12.0188747157874;93.5956721852260,13.3766506423594;93.5940862324273,14.4893551259315;93.5922498660288,15.7777497911201;93.6467565595843,17.5358535925655;93.7011797819399,19.3525207878831;93.6998442427410,20.2895350898385;93.6404962195894,21.9281081329814;93.6394945651902,22.6308688594480;93.5805638980383,23.9766249332299;93.6351540627938,25.6761653408030;93.5766407516415,26.7291044452238;93.6879078611507,28.6641004135649;93.6853202539528,30.4795656236035;93.6827326467549,32.2950308336420;93.8515948842171,33.8212850301566;93.8490072770192,35.6367502401952;93.9041817401742,36.9263468906629;94.0732943912362,38.2769109055608;94.0732943912362,38.2769109055608;94.0732943912362,38.2769109055608;94.0732943912362,38.2769109055608;94.0732943912362,38.2769109055608;94.0732943912362,38.2769109055608;94.0732943912362,38.2769109055608;94.0732943912362,38.2769109055608];
Traj_J = [55.0683213208573,36.9276993984038;55.0683213208573,36.9276993984038;55.0683213208573,36.9276993984038;55.0683213208573,36.9276993984038;55.0683213208573,36.9276993984038;55.0683213208573,36.9276993984038;55.0683213208573,36.9276993984038;55.0683213208573,36.9276993984038;55.0683213208573,36.9276993984038;55.0683213208573,36.9276993984038;55.0683213208573,36.9276993984038;55.1007320204605,36.5035860956944;55.1331427200636,36.0794727929849;55.1416773765218,35.6762102753343;55.1502120329801,35.2729477576837;55.1761069565521,34.8513745225409;55.2020018801242,34.4298012873981;55.2290606204861,33.9532377089393;55.2561193608479,33.4766741304805;55.2673695898155,32.9451008117592;55.2786198187832,32.4135274930380;55.2725097806370,31.9002648918088;55.2663997424907,31.3870022905797;55.3139222614058,30.7454870791195;55.3614447803209,30.1039718676592;55.3730829482184,29.5540684344992;55.3847211161160,29.0041650013393;55.3631905055055,28.4175625454090;55.3416598948950,27.8309600894788;55.3548498185122,27.2077361985642;55.3680397421295,26.5845123076495;55.4147863831847,25.9796573250666;55.4615330242399,25.3748023424836;55.4731711921375,24.8248989093237;55.4848093600351,24.2749954761638;55.5623971460188,23.8168202029831;55.6399849320026,23.3586449298025;55.6678195502243,22.8454211224664;55.6956541684459,22.3321973151302;55.7412369927114,21.7823326758633;55.7868198169769,21.2324680365963;55.8000097405941,20.6092441456817;55.8131996642113,19.9860202547671;55.8228981374593,19.5277673938005;55.8325966107073,19.0695145328339;55.8257106947012,18.5929121604821;55.8188247786952,18.1163097881303;55.8320147023124,17.4930858972157;55.8452046259296,16.8698620063011;55.8568427938272,16.3199585731412;55.8684809617248,15.7700551399812;55.8986432135260,15.1468506460131;55.9288054653272,14.5236461520450;55.9539245110394,14.1387331457795;55.9790435567516,13.7538201395141;55.9354974118683,13.4054897743400;55.8919512669849,13.0571594091658;55.9124150455381,12.8922077761644;55.9328788240913,12.7272561431629;55.8723603510240,12.3789063810423;55.8118418779566,12.0305566189217;55.7474440155901,11.8655080011877;55.6830461532236,11.7004593834537;55.6360085579709,11.5171000482276;55.5889709627183,11.3337407130014;55.5754900849036,11.1687502861070;55.5620092070889,11.0037598592125;55.4995510393720,10.7470606692852;55.4370928716550,10.4903614793579;55.2774560019934,10.0135845344876;55.1494361551202,9.64682707014238;54.9195823391433,9.27995322411814;54.6928320346058,8.76643846258459;54.3974165394726,8.28950634214237;54.0009429530955,7.77579761114385;53.7363686028909,7.44554520010396;53.4710183748264,7.15195301794139;53.1717234903940,6.85832204188582;52.9395420408376,6.60142888249357;52.4404586074970,6.12426399869340;52.1434913566441,5.72065233600585;51.9089822735082,5.57373986324559;51.6089115112160,5.31676911606735;51.1691827341530,5.24294433770380;50.7988950255455,5.09587668937157;50.4000000000000,5.02000000000000;50,4.95000000000000;49.6154873198281,4.87455752985288;49.1402621306775,4.87401441535099;48.7305986206832,4.98352957526708;48.2300000000000,5.10000000000000;47.6397143497515,5.20224954395531;46.9191177874272,5.56803716097578;46.4068444304694,5.71409616809023;45.6515273339174,6.11650522009503;45.4100353500430,6.29953480723074;44.9100000000000,6.65000000000000;44.4101227581772,7.03161436188056;43.9626352025158,7.32439187229031;43.2732548597340,7.82820889044432;42.9229460060173,8.34106415579702;42.7115192892115,8.70743368121236;42.5988230300701,9.22056050381600;42.3881721911242,9.55026980035402;42.1736419628790,10.0632802412787;41.9629911239331,10.3929895378167;41.9228394446865,10.6862325749423;41.8471913533523,11.0527572759297;41.8749289868415,11.3460779008413;41.8702737196825,11.5660392741053;41.8285702847162,11.9326027689856;41.8223632618375,12.2258846000042;41.8091733382203,12.8491084909188;41.8091733382203,12.8491084909188;41.8091733382203,12.8491084909188;41.8091733382203,12.8491084909188;41.8091733382203,12.8491084909188;41.8091733382203,12.8491084909188;41.8091733382203,12.8491084909188;41.8091733382203,12.8491084909188;41.8091733382203,12.8491084909188];

% Y=38, Z-6mm; Y = 4.8, Z+0mm;
height1_bias_Z = zeros(1,length(Traj_Z))';
height1_bias_J = zeros(1,length(Traj_J))';
height1_bias_U = zeros(1,length(Traj_U))';
height1_bias_Z = height1_bias_Z-0.006*(Traj_Z(:,2)-4.8)/(38-4.8);
height1_bias_J = height1_bias_J-0.006*(Traj_J(:,2)-4.8)/(38-4.8);
height1_bias_U = height1_bias_U-0.006*(Traj_U(:,2)-4.8)/(38-4.8);
% ind=1, Z+0mm; ind=end, Z+2mm
height1_bias_Z = height1_bias_Z+0.002*(0:length(Traj_Z)-1)'/(length(Traj_Z)-1);
height1_bias_J = height1_bias_J+0.002*(0:length(Traj_J)-1)'/(length(Traj_J)-1);
height1_bias_U = height1_bias_U+0.002*(0:length(Traj_U)-1)'/(length(Traj_U)-1);

Traj_Z(:,1) = (Traj_Z(:,1)-50)*scale_factor + Xcenter;
Traj_J(:,1) = (Traj_J(:,1)-50)*scale_factor + Xcenter;
Traj_U(:,1) = (Traj_U(:,1)-50)*scale_factor + Xcenter;
Traj_Z(:,2) = (Traj_Z(:,2)-20)*scale_factor + Ycenter;
Traj_J(:,2) = (Traj_J(:,2)-20)*scale_factor + Ycenter;
Traj_U(:,2) = (Traj_U(:,2)-20)*scale_factor + Ycenter;

% Z的轨迹
len1 = length(Traj_Z(:,1));
Traj1 = [Traj_Z,(height1 + height1_bias_Z).*ones(len1,1)];

% Z到J间的抬起轨迹
len2 = 40;
% Traj2 = [linspace(Traj_Z(end,1), Traj_J(1,1),len2)', linspace(Traj_Z(end,2), Traj_J(1,2),len2)', height2*ones(len2,1)];
Traj_up = [Traj_Z(end,1)*ones(10,1), Traj_Z(end,2)*ones(10,1), linspace(height1, height2,10)'];
Traj_down = [Traj_J(1,1)*ones(25,1), Traj_J(1,2)*ones(25,1), linspace(height2, height1,25)'];
Traj_tran = [linspace(Traj_Z(end,1), Traj_J(1,1),len2)', linspace(Traj_Z(end,2), Traj_J(1,2),len2)', height2*ones(len2,1)];
Traj2 = [Traj_up; Traj_tran; Traj_down];
len2 = len2+35;

% J的轨迹
len3 = length(Traj_J(:,1));
Traj3 = [Traj_J,(height1 + height1_bias_J).*ones(len3,1)];

% J到U间的抬起轨迹
len4 = 40;
Traj_up = [Traj_J(end,1)*ones(10,1), Traj_J(end,2)*ones(10,1), linspace(height1, height2,10)'];
Traj_down = [Traj_U(1,1)*ones(25,1), Traj_U(1,2)*ones(25,1), linspace(height2, height1,25)'];
Traj_tran = [linspace(Traj_J(end,1), Traj_U(1,1),len4)', linspace(Traj_J(end,2), Traj_U(1,2),len4)', height2*ones(len4,1)];
Traj4 = [Traj_up; Traj_tran; Traj_down];
len4 = len4+35;

% U的轨迹
len5 = length(Traj_U(:,1));
Traj5 = [Traj_U,(height1 + height1_bias_U).*ones(len5,1)];

% U回到Z间的抬起轨迹
len6 = 40;
% Traj6 = [linspace(Traj_U(end,1), Traj_Z(1,1),len6)', linspace(Traj_U(end,2), Traj_Z(1,2),len6)', height2*ones(len6,1)];
Traj_up = [Traj_U(end,1)*ones(10,1), Traj_U(end,2)*ones(10,1), linspace(height1, height2,10)'];
Traj_down = [Traj_Z(1,1)*ones(25,1), Traj_Z(1,2)*ones(25,1), linspace(height2, height1,25)'];
Traj_tran = [linspace(Traj_U(end,1), Traj_Z(1,1),len6)', linspace(Traj_U(end,2), Traj_Z(1,2),len6)', height2*ones(len6,1)];
Traj6 = [Traj_up; Traj_tran; Traj_down];
len6 = len6+35;

% 各段时间
% draw_time = span(1);
% suspend_time = span(2);
tick1 = span(1)/(len1-1);
tick2 = span(2)/(len2-1);
tick3 = span(3)/(len3-1);
tick4 = span(4)/(len4-1);
tick5 = span(5)/(len5-1);
tick6 = span(6)/(len6-1);

% 根据时间输出当前期望位置
err = 0;
if phase-phase_last == 1 || phase-phase_last == -6 % 新一段轨迹
	phase_start_time = time;
elseif phase-phase_last == 0
	phase_start_time = phase_start_time_last;
else
	phase_start_time = phase_start_time_last;
	err = 1;
end
traj = nan(1,3);
switch phase
	case 0
		traj = Traj1(1,:);
	case 1
		ind = max([1,ceil((time-phase_start_time)/tick1)]);
		ind = min([ind, len1]);
		traj = Traj1(ind,:);
	case 2
		ind = max([1,ceil((time-phase_start_time)/tick2)]);
		ind = min([ind, len2]);
		traj = Traj2(ind,:);
	case 3
		ind = max([1,ceil((time-phase_start_time)/tick3)]);
		ind = min([ind, len3]);
		traj = Traj3(ind,:);
	case 4
		ind = max([1,ceil((time-phase_start_time)/tick4)]);
		ind = min([ind, len4]);
		traj = Traj4(ind,:);
	case 5
		ind = max([1,ceil((time-phase_start_time)/tick5)]);
		ind = min([ind, len5]);
		traj = Traj5(ind,:);
	case 6
		ind = max([1,ceil((time-phase_start_time)/tick6)]);
		ind = min([ind, len6]);
		traj = Traj6(ind,:);
end
if max(isnan(traj))==1
	err = 2;
end

== matlab function RBFNN_1221/Subsystem9/MATLAB Function3 ==
  data: span input; y output; t input; reset input; t_terminal output; t_terminal_last input
function [y,t_terminal] = fcn(span, t, reset,t_terminal_last)
t_terminal=t_terminal_last;
if reset == 1
t_terminal = t;
end
t= t-t_terminal;

y = 0;
if t>=6
    y=1;
end
if t>=6+sum(span(1:1))
    y=2;
end
if t>=6+sum(span(1:2))
    y=3;
end
if t>=6+sum(span(1:3))
    y=4;
end
if t>=6+sum(span(1:4))
    y=5;
end
if t>=6+sum(span(1:5))
    y=6;
end

== matlab function RBFNN_1221/Subsystem9/Subsystem/B-Spline Traj Plan ==
  data: CtrlP output size=4,4; CtrlP_last input; pos output size=4,1; dpos output size=4,1; ddpos output; dddpos output; CtrlP_new input; clock input; sect_n_last input; sect_n output size=1; err output size=1; temp output
% B样条曲线轨迹规划函数(Simulink)
% 
% 功能
% 以20Hz速率读取前一模块规划的控制点，并更新B样条轨迹
% 
% 输入
% CtrlP_last：之前一个迭代中使用的几个控制点
% CtrlP_new：最新的控制点
% clock：时钟时间
% sect_n_last：上一迭代中，轨迹属于第几段
%
% 输出
% pos：规划得到的当前时刻轨迹位置
% CtrlP：当前使用的控制点
% sect_n：当前轨迹属于第几段
% err：模块报错信息
% temp：debug用的

function [CtrlP, pos, dpos, ddpos, dddpos, sect_n, err, temp] = fcn(CtrlP_last, CtrlP_new, clock, sect_n_last)

dim = 4; % 四维曲线
Ts = 1/30; % 控制点更新时间
pos = zeros(dim,1);
err = 0;
sect_n = floor(clock/Ts); % 本段轨迹属于第几段
t = mod(clock, Ts); % 本段轨迹已经历的时间
u = t; % B样条参数u=t
u = 3/9 + t/Ts/9;
k = 3; % 阶数 k
n = 2*(k+1); % 所需点数 n = 2 * (k+1) % 实际用到值的点数 k+1 (余下的点用0代替)
m = n+k+1; % m = n + k + 1
knots = linspace(0, 1, n+2); % 节点向量
% knots = linspace(0, 1, 10); % 节点向量
CtrlP = zeros(dim, k+1);
if sect_n_last == 0
	CtrlP_last = CtrlP;
end
if sect_n_last - sect_n == -1 % 新一段轨迹
	CtrlP = [CtrlP_last(:,2:end), CtrlP_new]; % 更新控制点
elseif sect_n_last - sect_n == 0 % 同一段轨迹
	CtrlP = CtrlP_last; % 不更新控制点
else
	err = -1;
end
CtrlP_extend = [CtrlP, zeros(dim, k+1)]; % 控制点补零
% pos = CtrlP(:,1);
for iP = 1:k+1
	pos = pos + BaseFunction(iP,k,u,knots) * CtrlP(:,iP);
% 	pos = CtrlP_extend(:,1);
end

dpos = zeros(dim,1);
CtrlQ = diff(CtrlP,1,2);
for iQ = 1:k
	CtrlQ(:,iQ) = k * CtrlQ(:,iQ) / (knots(iQ+k+1)-knots(iQ+1));
end
for iQ = 1:k
	dpos = dpos + BaseFunction(iQ+1, k-1, u, knots) * CtrlQ(:,iQ);
end
dpos = dpos /9/Ts;

k = k-1;
ddpos = zeros(dim,1);
CtrlR = diff(CtrlQ,1,2);
for iR = 1:k
	CtrlR(:,iR) = k * CtrlR(:,iR) / (knots(iR+k+1)-knots(iR+1));
end
for iR = 1:k
	ddpos = ddpos + BaseFunction(iR+2, k-1, u, knots) * CtrlR(:,iR);
end
ddpos = ddpos /3/Ts / 0.9;

k = k-1;
dddpos = zeros(dim,1);
CtrlS = diff(CtrlR,1,2);
for iS = 1:k
	CtrlS(:,iS) = k * CtrlS(:,iS) / (knots(iS+k+1)-knots(iS+1));
end
for iS = 1:k
	dddpos = dddpos + BaseFunction(iS+3, k-1, u, knots) * CtrlS(:,iS);
end
dddpos = dddpos /1/Ts /0.81;

temp = sect_n_last - sect_n;

== matlab function RBFNN_1221/Subsystem9/Subsystem/Control Point Plan ==
  data: CtrlP_last input size=4,1; Pf input size=4,1; p_init input; CtrlP output size=4,1; clock input size=1
% 路径控制点生成函数(Simulink)
% 
% 功能
% 依据之前模块得到的目标位置，以20Hz以上的速率更新路径控制点
%
% 输入
% CtrlP_last：上一次迭代用的控制点
% Pf：最终期望达到的位置
% p_init：初始位置，在第一次更新控制点前CtrlP_last=p_init
% clock：时钟时间
%
% 输出
% CtrlP：本次迭代控制点

function CtrlP = fcn(CtrlP_last, Pf, p_init, clock)

% CtrlP = 0.1*clock*ones(4,1);
% CtrlP = ones(4,1) * Pf;
vm = 0.05;
Ts = 0.02;
if clock <= Ts
	CtrlP = [-0.1; 0.8; -0.3; 0];
	return
end
if mod(clock, Ts) <= 0.2e-3
	step_max = vm*Ts;
	dis = Pf - CtrlP_last;
	dis = sqrt(sum(dis.^2));
	if dis ~= 0
		dir = (Pf - CtrlP_last) / dis;
		k = 2/step_max;
		CtrlP = CtrlP_last + dir * step_max * (1-exp(-k*dis)) / (1+exp(-k*dis));
	else
		CtrlP = CtrlP_last;
	end
else
	CtrlP = CtrlP_last;
end
if clock < Ts
	CtrlP = p_init;
end

== matlab function RBFNN_1221/Subsystem9/Subsystem/Inverse Kinematics ==
  data: pos_obj input; pos_relative input; q_f output
function q_f = fcn(pos_obj, pos_relative)

% if mod(clock, Ts) <= 0.2e-3
% pos_relative = [0;0;-0.1];
q_f = InvKin(pos_relative, pos_obj);

end

== matlab function RBFNN_1221/Subsystem9/MATLAB Function2 ==
  data: q input; y output
function y = fcn(q)
p = FK(q,[0,0,-1]);
y = p(1:3);

== matlab function RBFNN_1221/q2qfdot_rad ==
  data: ts input; qf_next output; q input; qf input; qf_dot input; qf_dot_next output
function [qf_next, qf_dot_next] = q2qfdot_rad(ts, q, qf, qf_dot)

wn = 50;% 为了减少相位滞后，应尽可能大，但是过大会受到噪声的影响
epsilon = 0.707;


qf_ddot = wn^2*(q-qf) - 2*wn*epsilon*qf_dot;
qf_dot_next = qf + qf_ddot.*ts;
qf_next = qf + qf_dot.*ts;
